simulink model "chap9_5sim"  (Simulink 3.00)
settings: Solver=ode5  StartTime=0.0  StopTime=3  FixedStep=0.001  RelTol=1e-3
settings Model: LastModifiedBy=liu

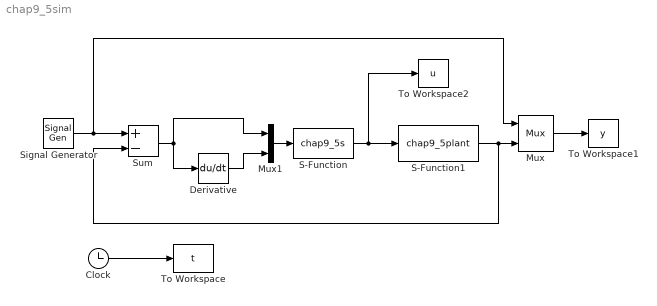
== system chap9_5sim ==
  Clock : Clock
      settings: DisplayTime=off  Decimation=10
  Derivative : Derivative
  Mux : Mux  Inputs=2
      settings: DisplayOption=none
  Mux1 : Mux  Inputs=2
  S-Function : S-Function  FunctionName=chap9_5s  PortCounts=[]  SFunctionModules=''
  S-Function1 : S-Function  FunctionName=chap9_5plant  PortCounts=[]  SFunctionModules=''
  Signal Generator : SignalGenerator  WaveForm=sine  Amplitude=1  Frequency=3  Units=Hertz
  Sum : Sum  Inputs=+-  SaturateOnIntegerOverflow=on
  To Workspace : ToWorkspace  VariableName=t  SampleTime=-1  SaveFormat=Matrix
  To Workspace1 : ToWorkspace  VariableName=y  SampleTime=-1  SaveFormat=Matrix
  To Workspace2 : ToWorkspace  VariableName=u  SampleTime=-1  SaveFormat=Matrix
  wires:
  Clock/1 -> To Workspace/1
  Mux1/1 -> S-Function/1
  Derivative/1 -> Mux1/2
  Mux/1 -> To Workspace1/1
  S-Function1/1 -> Mux/2, Sum/2
  S-Function/1 -> S-Function1/1, To Workspace2/1
  Sum/1 -> Derivative/1, Mux1/1
  Signal Generator/1 -> Sum/1, Mux/1
